simulink model "penultimolabdelabida"  (R2018a)
settings: Solver=VariableStepAuto  StartTime=0.0  StopTime=30  RelTol=1e-3
values from neighbouring files (symbols this model uses):
  A_0 = [0 -3.26931291643 0 0.71460251427 0 0 0 0 1 -0.0325743287495 0 -0.000548520916999 ... (64 elements, 8x8)]    [parametros.mat]    (also in twin_rotor_modelo_V1.m = eval(A_0))
  B_0 = [0 0 0 0 0 0 1190.47619048 0 0 0 0 0 ... (16 elements, 8x2)]    [parametros.mat]    (also in twin_rotor_modelo_V1.m = eval(B_0))
  C_0 = [1 0 0 0 0 1 0 0 0 0 0 0 ... (16 elements, 2x8)]    [parametros.mat]    (also in twin_rotor_modelo_V1.m = eval(C_0))
  Q = [ ... (first row only)    [ele_cu_erre_para_iterar.m]    (also in elecuerre.m)
  R = [ ... (first row only)    [ele_cu_erre_para_iterar.m]    (also in elecuerre.m; twin_rotor_modelo_V1.m = R2*R1)
  u0 = [11.9668031953 -0.0853053139382]    [parametros.mat]    (also in twin_rotor_modelo_V1.m = [u_p_0;u_t_0])
undefined symbols (not defined in the file or in its folder): K
settings Model: Creator=Gonzalo  LastModifiedBy=Gonzalo

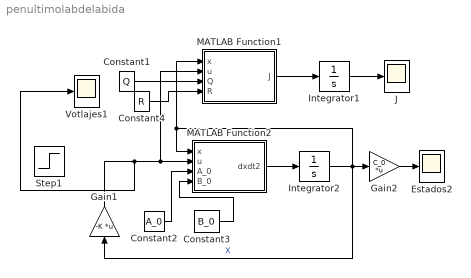
== system penultimolabdelabida ==
  Constant1 : Constant  Value=Q
  Constant2 : Constant  Value=A_0
  Constant3 : Constant  Value=B_0
  Constant4 : Constant  Value=R
  Estados2 : Scope
  Gain1 : Gain  Gain=-K  Multiplication=Matrix(K*u)
  Gain2 : Gain  Gain=C_0  Multiplication=Matrix(K*u)
  Integrator1 : Integrator  InitialCondition=[pi/6 0 0 0 0 0 0 0]
  Integrator2 : Integrator  InitialCondition=[pi/6 0 0 0 0 0 0 0]
  J : Scope
  MATLAB Function1 : MATLAB Function  TreatAsAtomicUnit=on
  MATLAB Function2 : MATLAB Function  TreatAsAtomicUnit=on
  Step1 : Step  Time=10  Before=u0  After=u0  SampleTime=0
  Votlajes1 : Scope
  wires:
  Constant2/1 -> MATLAB Function2/3(A_0)
  Constant3/1 -> MATLAB Function2/4(B_0)
  Gain2/1 -> Estados2/1
  Integrator2/1 -> Gain1/1, MATLAB Function1/1(x), MATLAB Function2/1(x), Gain2/1  "X"
  MATLAB Function2/1(dxdt2) -> Integrator2/1
  Gain1/1 -> Votlajes1/1, MATLAB Function2/2(u), MATLAB Function1/2(u)
  Constant1/1 -> MATLAB Function1/3(Q)
  Constant4/1 -> MATLAB Function1/4(R)
  MATLAB Function1/1(J) -> Integrator1/1
  Integrator1/1 -> J/1

== matlab function penultimolabdelabida/MATLAB Function1 ==
  data: x input; u input; J output; Q input; R input
function J = funcion(x,u,Q,R)
J = x'*Q*x + u'*R*u;

== matlab function penultimolabdelabida/MATLAB Function2 ==
  data: x input; u input; dxdt2 output; A_0 input; B_0 input
function dxdt2 = funcion(x,u,A_0,B_0)
dxdt2 = A_0*x + B_0*u;
